simulink model "SGBMDisparityExample_original"  (R2021a)
settings: Solver=FixedStepDiscrete  StartTime=0.0  StopTime=simT  FixedStep=1  RelTol=1e-3
PreLoadFcn:
  | DL128 = Simulink.Variant('disparityLevels==128');
  | 
  | DLnot128 = Simulink.Variant('disparityLevels ~= 128');
  | 
  | disparityLevels = 64;
  | 
  | imgRowSize = 480;
  | 
  | imgColSize = 640;
  | 
  | P2 = 200; % Smoothness Penalty Large
  | P1 = 15;  % Smoothness Penalty Small
  | 
  | disparityFactor = 16;
  | 
  | uniquenessRatio = 5;
  | 
  | p = imgColSize - 1;
  | q = imgRowSize * imgColSize -1;
  | r = imgColSize - disparityLevels -1;
  | s = (imgRowSize*(imgColSize-disparityLevels))-1;
  | 
  | simT = 800*525
  | 
  | dtGain = 4;
InitFcn:
  | DL128 = Simulink.Variant('disparityLevels==128');
  | 
  | DLnot128 = Simulink.Variant('disparityLevels ~= 128');
  | 
  | img = imread(get_param('SGBMDisparityExample/leftImage','FileName'));
  | 
  | [imgRowSize, imgColSize] = size(img);
  | 
  | P2 = 200; % Smoothness Penalty Large
  | P1 = 15;  % Smoothness Penalty Small
  | 
  | disparityFactor = 16;
  | 
  | uniquenessRatio = str2num(get_param('SGBMDisparityExample/SGBMHDLAlgorithm','UT'));
  | 
  | disparityLevels = str2num(get_param('SGBMDisparityExample/SGBMHDLAlgorithm','DL'));
  | 
  | p = imgColSize - 1;
  | q = imgRowSize * imgColSize -1;
  | r = imgColSize - disparityLevels -1;
  | s = (imgRowSize*(imgColSize-disparityLevels))-1;
  | 
  | if imgRowSize == 720 && imgColSize == 1280
  | simT = 1650*750;
  | elseif imgRowSize == 540 && imgColSize == 960
  | simT = 1050*600;
  | elseif imgRowSize == 480 && imgColSize == 640
  | simT = 800*525;
  | end
  | 
  | if imgRowSize == 720 && imgColSize == 1280
  | dtGain = 2;
  | elseif imgRowSize == 540 && imgColSize == 960
  | dtGain = 2.6;
  | elseif imgRowSize == 480 && imgColSize == 640
  | dtGain = 4;
  | end
libraries: simulink x331, hdlsllib x105, visionhdlutilities x10, visionhdlio x4, visionsources x3
(part 5 of 6)

== system SGBMDisparityExample_original/SGBMHDLAlgorithm/MatchingCost/CensusTransform1/validLogic/pixelBusGenerator ==
  validIn : Inport
  Horizontal : hdlsllib/Sources/HDL Counter  CountType=Count limited  CountInit=0  CountStep=1  CountMax=hEnd  CountFromType=Initial value  CountFrom=0  CountResetPort=off  CountLoadPort=off  CountEnbPort=on  CountDirPort=off  CountHitOutputPort=off  CountDataType=Unsigned  CountWordLen=ceil(log2(hEnd))  CountFracLen=0  CountSampTime=1
  Logical Operator{3..6} (4 alike) : Logic  AllPortsSameDT=off  OutDataTypeStr=boolean
  Pixel Control Bus Creator : visionhdlutilities/Pixel Control Bus Creator
      settings: SourceProductBaseCode=VT
  Vertical : hdlsllib/Sources/HDL Counter  CountType=Count limited  CountInit=0  CountStep=1  CountMax=vEnd  CountFromType=Initial value  CountFrom=0  CountResetPort=off  CountLoadPort=off  CountEnbPort=on  CountDirPort=off  CountHitOutputPort=off  CountDataType=Unsigned  CountWordLen=ceil(log2(vEnd))  CountFracLen=0  CountSampTime=1
  hEnd : simulink/Logic and Bit Operations/Compare To Constant  relop===  const=hEnd  OutDataTypeStr=boolean
  hStart : simulink/Logic and Bit Operations/Compare To Constant  relop===  const=0  OutDataTypeStr=boolean
  vEnd : simulink/Logic and Bit Operations/Compare To Constant  relop===  const=vEnd  OutDataTypeStr=boolean
  vStart : simulink/Logic and Bit Operations/Compare To Constant  relop===  const=0  OutDataTypeStr=boolean
  busOut : Outport  VectorParamsAs1DForOutWhenUnconnected=off
  wires:
  validIn/1 -> Pixel Control Bus Creator/5, Vertical/1, Logical Operator4/1, Logical Operator5/1, Logical Operator6/1, Logical Operator3/1, Horizontal/1
  Horizontal/1 -> hEnd/1, hStart/1
  hEnd/1 -> Logical Operator4/2
  Vertical/1 -> vStart/1, vEnd/1
  vStart/1 -> Logical Operator5/2
  vEnd/1 -> Logical Operator6/2
  Logical Operator5/1 -> Pixel Control Bus Creator/3
  Logical Operator3/1 -> Pixel Control Bus Creator/1
  Logical Operator4/1 -> Pixel Control Bus Creator/2
  hStart/1 -> Logical Operator3/2
  Logical Operator6/1 -> Pixel Control Bus Creator/4
  Pixel Control Bus Creator/1 -> busOut/1

== system SGBMDisparityExample_original/SGBMHDLAlgorithm/MatchingCost/CensusTransform1/zeroPadding/FIFO ==
  dataIn : Inport
  Push : Inport  Port=2
  Pop : Inport  Port=3
  Reset : Inport  Port=4
  EmpltyFlag : RelationalOperator  Operator===  OutDataTypeStr=boolean  RndMeth=Nearest
  HDL Counter : hdlsllib/Sources/HDL Counter  CountType=Count limited  CountInit=0  CountStep=1  CountMax=((imgRowSize+6)*(imgColSize+8))-(imgRowSize*imgColSize)  CountFromType=Initial value  CountFrom=0  CountResetPort=on  CountLoadPort=off  CountEnbPort=on  CountDirPort=off  CountHitOutputPort=off  CountDataType=Unsigned  CountWordLen=ceil(log2(((imgRowSize+6)*(imgColSize+8))-(imgRowSize*imgColSize)))  CountFracLen=0  CountSampTime=1
  HDL Counter1 : hdlsllib/Sources/HDL Counter  CountType=Count limited  CountInit=0  CountStep=1  CountMax=((imgRowSize+6)*(imgColSize+8))-(imgRowSize*imgColSize)  CountFromType=Initial value  CountFrom=0  CountResetPort=on  CountLoadPort=off  CountEnbPort=on  CountDirPort=off  CountHitOutputPort=off  CountDataType=Unsigned  CountWordLen=ceil(log2(((imgRowSize+6)*(imgColSize+8))-(imgRowSize*imgColSize)))  CountFracLen=0  CountSampTime=1
  Simple Dual Port RAM : hdlsllib/HDL RAMs/Simple Dual Port RAM  ram_size=ceil(log2(((imgRowSize+6)*(imgColSize+8))-(imgRowSize*imgColSize)))
      settings: SourceProductBaseCode=SL
  dataOut : Outport  VectorParamsAs1DForOutWhenUnconnected=off
  empty : Outport  Port=2  VectorParamsAs1DForOutWhenUnconnected=off
  wires:
  HDL Counter1/1 -> EmpltyFlag/2, Simple Dual Port RAM/4
  Pop/1 -> HDL Counter1/2
  HDL Counter/1 -> EmpltyFlag/1, Simple Dual Port RAM/2
  Push/1 -> HDL Counter/2, Simple Dual Port RAM/3
  dataIn/1 -> Simple Dual Port RAM/1
  Simple Dual Port RAM/1 -> dataOut/1
  EmpltyFlag/1 -> empty/1
  Reset/1 -> HDL Counter1/1, HDL Counter/1

== system SGBMDisparityExample_original/SGBMHDLAlgorithm/MatchingCost/CensusTransform1/zeroPadding/popSubsystem ==
  enable : Inport
  reset : Inport  Port=2
  Enable : EnablePort
  CC : simulink/Logic and Bit Operations/Compare To Constant  relop===  const=imgColSize+7  OutDataTypeStr=boolean
  CC1 : simulink/Logic and Bit Operations/Compare To Constant  relop=>=  const=3  OutDataTypeStr=boolean
  CC2 : simulink/Logic and Bit Operations/Compare To Constant  relop=>=  const=4  OutDataTypeStr=boolean
  CC3 : simulink/Logic and Bit Operations/Compare To Constant  relop=<  const=imgColSize+4  OutDataTypeStr=boolean
  CC4 : simulink/Logic and Bit Operations/Compare To Constant  relop=<  const=imgRowSize + 3  OutDataTypeStr=boolean
  CC6 : simulink/Logic and Bit Operations/Compare To Constant  relop===  const=imgRowSize + 5  OutDataTypeStr=boolean
  CC8 : simulink/Logic and Bit Operations/Compare To Constant  relop=>=  const=imgRowSize+2  OutDataTypeStr=boolean
  HDLC1 : hdlsllib/Sources/HDL Counter  CountType=Count limited  CountInit=0  CountStep=1  CountMax=imgColSize+7  CountFromType=Initial value  CountFrom=0  CountResetPort=on  CountLoadPort=off  CountEnbPort=on  CountDirPort=off  CountHitOutputPort=off  CountDataType=Unsigned  CountWordLen=ceil(log2(imgColSize+7))  CountFracLen=0  CountSampTime=1
  HDLC2 : hdlsllib/Sources/HDL Counter  CountType=Count limited  CountInit=0  CountStep=1  CountMax=imgRowSize+6  CountFromType=Initial value  CountFrom=0  CountResetPort=on  CountLoadPort=off  CountEnbPort=on  CountDirPort=off  CountHitOutputPort=off  CountDataType=Unsigned  CountWordLen=ceil(log2(imgRowSize+6))  CountFracLen=0  CountSampTime=1
  LO2 : Logic  Inputs=4  AllPortsSameDT=off  OutDataTypeStr=boolean
  LO4 : Logic  AllPortsSameDT=off  OutDataTypeStr=boolean
  done : Outport  InitialOutput=0  VectorParamsAs1DForOutWhenUnconnected=off
  pop : Outport  Port=2  InitialOutput=0  VectorParamsAs1DForOutWhenUnconnected=off
  lastRowOut : Outport  Port=3  InitialOutput=0  VectorParamsAs1DForOutWhenUnconnected=off
  wires:
  HDLC2/1 -> CC1/1, CC6/1, CC8/1, CC4/1
  CC4/1 -> LO2/2
  HDLC1/1 -> CC3/1, CC2/1, CC/1
  CC/1 -> HDLC2/2, LO4/1
  CC2/1 -> LO2/3
  CC3/1 -> LO2/4
  CC1/1 -> LO2/1
  CC6/1 -> LO4/2
  LO2/1 -> pop/1
  CC8/1 -> lastRowOut/1
  enable/1 -> HDLC1/2
  LO4/1 -> done/1
  reset/1 -> HDLC2/1, HDLC1/1

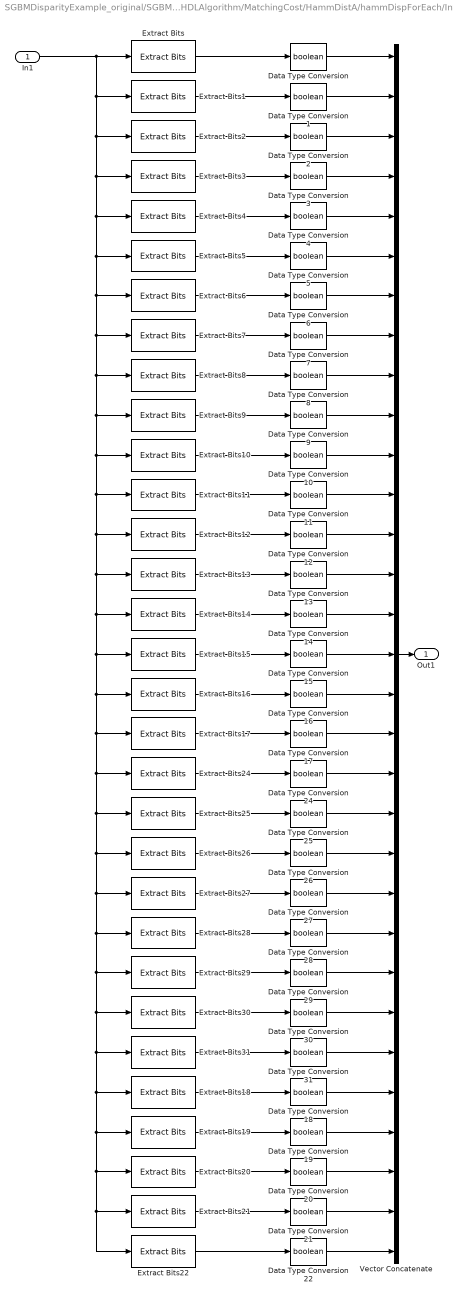
== system SGBMDisparityExample_original/SGBMHDLAlgorithm/MatchingCost/HammDistA/hammDispForEach/Int2Bin1 ==
  In1 : Inport
  Data Type Conversion{,1..22,24..31} (31 alike) : DataTypeConversion  OutDataTypeStr=boolean
  Extract Bits : simulink/Logic and Bit Operations/Extract Bits  bitsToExtract=Range of bits  numBits=8  bitIdxRange=[30]  outScalingMode=Treat bit field as an integer
  Extract Bits1 : simulink/Logic and Bit Operations/Extract Bits  bitsToExtract=Range of bits  numBits=8  bitIdxRange=[29]  outScalingMode=Treat bit field as an integer
  Extract Bits10 : simulink/Logic and Bit Operations/Extract Bits  bitsToExtract=Range of bits  numBits=8  bitIdxRange=[20]  outScalingMode=Preserve fixed-point scaling
  Extract Bits11 : simulink/Logic and Bit Operations/Extract Bits  bitsToExtract=Range of bits  numBits=8  bitIdxRange=[19]  outScalingMode=Preserve fixed-point scaling
  Extract Bits12 : simulink/Logic and Bit Operations/Extract Bits  bitsToExtract=Range of bits  numBits=8  bitIdxRange=[18]  outScalingMode=Preserve fixed-point scaling
  Extract Bits13 : simulink/Logic and Bit Operations/Extract Bits  bitsToExtract=Range of bits  numBits=8  bitIdxRange=[17]  outScalingMode=Preserve fixed-point scaling
  Extract Bits14 : simulink/Logic and Bit Operations/Extract Bits  bitsToExtract=Range of bits  numBits=8  bitIdxRange=[16]  outScalingMode=Preserve fixed-point scaling
  Extract Bits15 : simulink/Logic and Bit Operations/Extract Bits  bitsToExtract=Range of bits  numBits=8  bitIdxRange=[15]  outScalingMode=Preserve fixed-point scaling
  Extract Bits16 : simulink/Logic and Bit Operations/Extract Bits  bitsToExtract=Range of bits  numBits=8  bitIdxRange=[14]  outScalingMode=Preserve fixed-point scaling
  Extract Bits17 : simulink/Logic and Bit Operations/Extract Bits  bitsToExtract=Range of bits  numBits=8  bitIdxRange=[13]  outScalingMode=Preserve fixed-point scaling
  Extract Bits18 : simulink/Logic and Bit Operations/Extract Bits  bitsToExtract=Range of bits  numBits=8  bitIdxRange=[4]  outScalingMode=Preserve fixed-point scaling
  Extract Bits19 : simulink/Logic and Bit Operations/Extract Bits  bitsToExtract=Range of bits  numBits=8  bitIdxRange=[3]  outScalingMode=Preserve fixed-point scaling
  Extract Bits2 : simulink/Logic and Bit Operations/Extract Bits  bitsToExtract=Range of bits  numBits=8  bitIdxRange=[28]  outScalingMode=Treat bit field as an integer
  Extract Bits20 : simulink/Logic and Bit Operations/Extract Bits  bitsToExtract=Range of bits  numBits=8  bitIdxRange=[2]  outScalingMode=Preserve fixed-point scaling
  Extract Bits21 : simulink/Logic and Bit Operations/Extract Bits  bitsToExtract=Range of bits  numBits=8  bitIdxRange=[1]  outScalingMode=Preserve fixed-point scaling
  Extract Bits22 : simulink/Logic and Bit Operations/Extract Bits  bitsToExtract=Range of bits  numBits=8  bitIdxRange=[0]  outScalingMode=Preserve fixed-point scaling
  Extract Bits24 : simulink/Logic and Bit Operations/Extract Bits  bitsToExtract=Range of bits  numBits=8  bitIdxRange=[12]  outScalingMode=Preserve fixed-point scaling
  Extract Bits25 : simulink/Logic and Bit Operations/Extract Bits  bitsToExtract=Range of bits  numBits=8  bitIdxRange=[11]  outScalingMode=Preserve fixed-point scaling
  Extract Bits26 : simulink/Logic and Bit Operations/Extract Bits  bitsToExtract=Range of bits  numBits=8  bitIdxRange=[10]  outScalingMode=Preserve fixed-point scaling
  Extract Bits27 : simulink/Logic and Bit Operations/Extract Bits  bitsToExtract=Range of bits  numBits=8  bitIdxRange=[9]  outScalingMode=Preserve fixed-point scaling
  Extract Bits28 : simulink/Logic and Bit Operations/Extract Bits  bitsToExtract=Range of bits  numBits=8  bitIdxRange=[8]  outScalingMode=Preserve fixed-point scaling
  Extract Bits29 : simulink/Logic and Bit Operations/Extract Bits  bitsToExtract=Range of bits  numBits=8  bitIdxRange=[7]  outScalingMode=Preserve fixed-point scaling
  Extract Bits3 : simulink/Logic and Bit Operations/Extract Bits  bitsToExtract=Range of bits  numBits=8  bitIdxRange=[27]  outScalingMode=Treat bit field as an integer
  Extract Bits30 : simulink/Logic and Bit Operations/Extract Bits  bitsToExtract=Range of bits  numBits=8  bitIdxRange=[6]  outScalingMode=Preserve fixed-point scaling
  Extract Bits31 : simulink/Logic and Bit Operations/Extract Bits  bitsToExtract=Range of bits  numBits=8  bitIdxRange=[5]  outScalingMode=Preserve fixed-point scaling
  Extract Bits4 : simulink/Logic and Bit Operations/Extract Bits  bitsToExtract=Range of bits  numBits=8  bitIdxRange=[26]  outScalingMode=Treat bit field as an integer
  Extract Bits5 : simulink/Logic and Bit Operations/Extract Bits  bitsToExtract=Range of bits  numBits=8  bitIdxRange=[25]  outScalingMode=Treat bit field as an integer
  Extract Bits6 : simulink/Logic and Bit Operations/Extract Bits  bitsToExtract=Range of bits  numBits=8  bitIdxRange=[24]  outScalingMode=Treat bit field as an integer
  Extract Bits7 : simulink/Logic and Bit Operations/Extract Bits  bitsToExtract=Range of bits  numBits=8  bitIdxRange=[23]  outScalingMode=Treat bit field as an integer
  Extract Bits8 : simulink/Logic and Bit Operations/Extract Bits  bitsToExtract=Range of bits  numBits=8  bitIdxRange=[22]  outScalingMode=Preserve fixed-point scaling
  Extract Bits9 : simulink/Logic and Bit Operations/Extract Bits  bitsToExtract=Range of bits  numBits=8  bitIdxRange=[21]  outScalingMode=Preserve fixed-point scaling
  Vector Concatenate : Concatenate  NumInputs=31
  Out1 : Outport  VectorParamsAs1DForOutWhenUnconnected=off
  wires:
  Extract Bits6/1 -> Data Type Conversion6/1
  Extract Bits8/1 -> Data Type Conversion8/1
  Extract Bits1/1 -> Data Type Conversion1/1
  Extract Bits2/1 -> Data Type Conversion2/1
  Extract Bits9/1 -> Data Type Conversion9/1
  Extract Bits10/1 -> Data Type Conversion10/1
  Extract Bits3/1 -> Data Type Conversion3/1
  Extract Bits4/1 -> Data Type Conversion4/1
  Extract Bits11/1 -> Data Type Conversion11/1
  Extract Bits12/1 -> Data Type Conversion12/1
  Extract Bits13/1 -> Data Type Conversion13/1
  Extract Bits/1 -> Data Type Conversion/1
  Extract Bits7/1 -> Data Type Conversion7/1
  Extract Bits5/1 -> Data Type Conversion5/1
  Extract Bits31/1 -> Data Type Conversion31/1
  Extract Bits26/1 -> Data Type Conversion26/1
  Extract Bits18/1 -> Data Type Conversion18/1
  Extract Bits14/1 -> Data Type Conversion14/1
  Extract Bits21/1 -> Data Type Conversion21/1
  Extract Bits16/1 -> Data Type Conversion16/1
  Extract Bits25/1 -> Data Type Conversion25/1
  Extract Bits27/1 -> Data Type Conversion27/1
  Extract Bits30/1 -> Data Type Conversion30/1
  Extract Bits20/1 -> Data Type Conversion20/1
  Extract Bits28/1 -> Data Type Conversion28/1
  Extract Bits22/1 -> Data Type Conversion22/1
  Extract Bits24/1 -> Data Type Conversion24/1
  Extract Bits19/1 -> Data Type Conversion19/1
  Extract Bits15/1 -> Data Type Conversion15/1
  Extract Bits17/1 -> Data Type Conversion17/1
  Extract Bits29/1 -> Data Type Conversion29/1
  Vector Concatenate/1 -> Out1/1
  In1/1 -> Extract Bits/1, Extract Bits1/1, Extract Bits2/1, Extract Bits3/1, Extract Bits4/1, Extract Bits5/1, Extract Bits6/1, Extract Bits7/1, Extract Bits8/1, Extract Bits9/1, Extract Bits10/1, Extract Bits11/1, Extract Bits12/1, Extract Bits13/1, Extract Bits14/1, Extract Bits15/1, Extract Bits16/1, Extract Bits17/1, Extract Bits24/1, Extract Bits25/1, Extract Bits26/1, Extract Bits27/1, Extract Bits28/1, Extract Bits29/1, Extract Bits30/1, Extract Bits31/1, Extract Bits18/1, Extract Bits19/1, Extract Bits20/1, Extract Bits21/1, Extract Bits22/1
  Data Type Conversion/1 -> Vector Concatenate/1
  Data Type Conversion1/1 -> Vector Concatenate/2
  Data Type Conversion2/1 -> Vector Concatenate/3
  Data Type Conversion3/1 -> Vector Concatenate/4
  Data Type Conversion4/1 -> Vector Concatenate/5
  Data Type Conversion7/1 -> Vector Concatenate/8
  Data Type Conversion6/1 -> Vector Concatenate/7
  Data Type Conversion5/1 -> Vector Concatenate/6
  Data Type Conversion8/1 -> Vector Concatenate/9
  Data Type Conversion10/1 -> Vector Concatenate/11
  Data Type Conversion9/1 -> Vector Concatenate/10
  Data Type Conversion11/1 -> Vector Concatenate/12
  Data Type Conversion14/1 -> Vector Concatenate/15
  Data Type Conversion12/1 -> Vector Concatenate/13
  Data Type Conversion13/1 -> Vector Concatenate/14
  Data Type Conversion15/1 -> Vector Concatenate/16
  Data Type Conversion20/1 -> Vector Concatenate/29
  Data Type Conversion21/1 -> Vector Concatenate/30
  Data Type Conversion24/1 -> Vector Concatenate/19
  Data Type Conversion22/1 -> Vector Concatenate/31
  Data Type Conversion27/1 -> Vector Concatenate/22
  Data Type Conversion26/1 -> Vector Concatenate/21
  Data Type Conversion25/1 -> Vector Concatenate/20
  Data Type Conversion29/1 -> Vector Concatenate/24
  Data Type Conversion28/1 -> Vector Concatenate/23
  Data Type Conversion30/1 -> Vector Concatenate/25
  Data Type Conversion31/1 -> Vector Concatenate/26
  Data Type Conversion16/1 -> Vector Concatenate/17
  Data Type Conversion17/1 -> Vector Concatenate/18
  Data Type Conversion19/1 -> Vector Concatenate/28
  Data Type Conversion18/1 -> Vector Concatenate/27

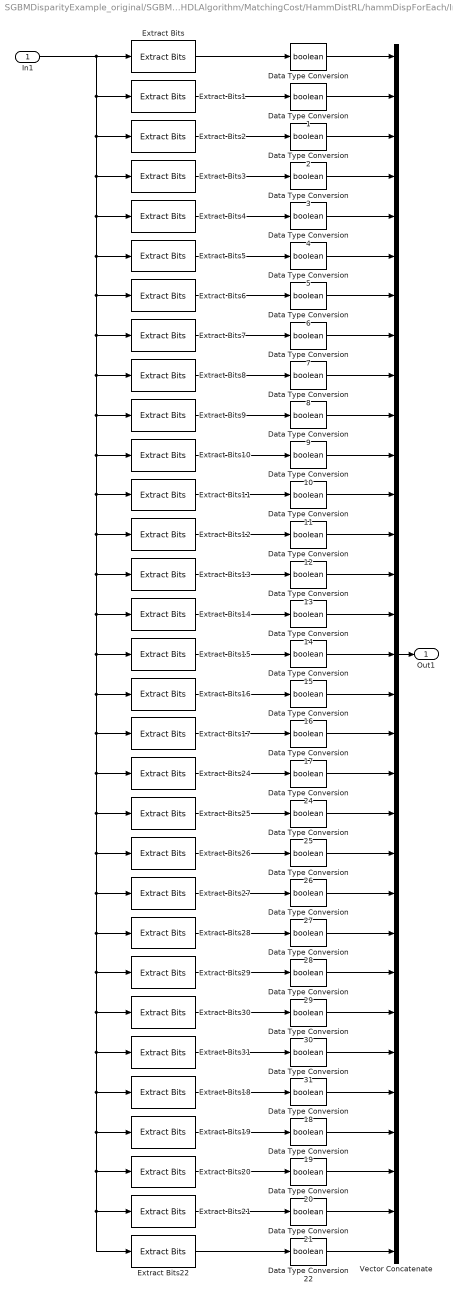
== system SGBMDisparityExample_original/SGBMHDLAlgorithm/MatchingCost/HammDistRL/hammDispForEach/Int2Bin1 ==
  In1 : Inport
  Data Type Conversion{,1..22,24..31} (31 alike) : DataTypeConversion  OutDataTypeStr=boolean
  Extract Bits : simulink/Logic and Bit Operations/Extract Bits  bitsToExtract=Range of bits  numBits=8  bitIdxRange=[30]  outScalingMode=Treat bit field as an integer
  Extract Bits1 : simulink/Logic and Bit Operations/Extract Bits  bitsToExtract=Range of bits  numBits=8  bitIdxRange=[29]  outScalingMode=Treat bit field as an integer
  Extract Bits10 : simulink/Logic and Bit Operations/Extract Bits  bitsToExtract=Range of bits  numBits=8  bitIdxRange=[20]  outScalingMode=Preserve fixed-point scaling
  Extract Bits11 : simulink/Logic and Bit Operations/Extract Bits  bitsToExtract=Range of bits  numBits=8  bitIdxRange=[19]  outScalingMode=Preserve fixed-point scaling
  Extract Bits12 : simulink/Logic and Bit Operations/Extract Bits  bitsToExtract=Range of bits  numBits=8  bitIdxRange=[18]  outScalingMode=Preserve fixed-point scaling
  Extract Bits13 : simulink/Logic and Bit Operations/Extract Bits  bitsToExtract=Range of bits  numBits=8  bitIdxRange=[17]  outScalingMode=Preserve fixed-point scaling
  Extract Bits14 : simulink/Logic and Bit Operations/Extract Bits  bitsToExtract=Range of bits  numBits=8  bitIdxRange=[16]  outScalingMode=Preserve fixed-point scaling
  Extract Bits15 : simulink/Logic and Bit Operations/Extract Bits  bitsToExtract=Range of bits  numBits=8  bitIdxRange=[15]  outScalingMode=Preserve fixed-point scaling
  Extract Bits16 : simulink/Logic and Bit Operations/Extract Bits  bitsToExtract=Range of bits  numBits=8  bitIdxRange=[14]  outScalingMode=Preserve fixed-point scaling
  Extract Bits17 : simulink/Logic and Bit Operations/Extract Bits  bitsToExtract=Range of bits  numBits=8  bitIdxRange=[13]  outScalingMode=Preserve fixed-point scaling
  Extract Bits18 : simulink/Logic and Bit Operations/Extract Bits  bitsToExtract=Range of bits  numBits=8  bitIdxRange=[4]  outScalingMode=Preserve fixed-point scaling
  Extract Bits19 : simulink/Logic and Bit Operations/Extract Bits  bitsToExtract=Range of bits  numBits=8  bitIdxRange=[3]  outScalingMode=Preserve fixed-point scaling
  Extract Bits2 : simulink/Logic and Bit Operations/Extract Bits  bitsToExtract=Range of bits  numBits=8  bitIdxRange=[28]  outScalingMode=Treat bit field as an integer
  Extract Bits20 : simulink/Logic and Bit Operations/Extract Bits  bitsToExtract=Range of bits  numBits=8  bitIdxRange=[2]  outScalingMode=Preserve fixed-point scaling
  Extract Bits21 : simulink/Logic and Bit Operations/Extract Bits  bitsToExtract=Range of bits  numBits=8  bitIdxRange=[1]  outScalingMode=Preserve fixed-point scaling
  Extract Bits22 : simulink/Logic and Bit Operations/Extract Bits  bitsToExtract=Range of bits  numBits=8  bitIdxRange=[0]  outScalingMode=Preserve fixed-point scaling
  Extract Bits24 : simulink/Logic and Bit Operations/Extract Bits  bitsToExtract=Range of bits  numBits=8  bitIdxRange=[12]  outScalingMode=Preserve fixed-point scaling
  Extract Bits25 : simulink/Logic and Bit Operations/Extract Bits  bitsToExtract=Range of bits  numBits=8  bitIdxRange=[11]  outScalingMode=Preserve fixed-point scaling
  Extract Bits26 : simulink/Logic and Bit Operations/Extract Bits  bitsToExtract=Range of bits  numBits=8  bitIdxRange=[10]  outScalingMode=Preserve fixed-point scaling
  Extract Bits27 : simulink/Logic and Bit Operations/Extract Bits  bitsToExtract=Range of bits  numBits=8  bitIdxRange=[9]  outScalingMode=Preserve fixed-point scaling
  Extract Bits28 : simulink/Logic and Bit Operations/Extract Bits  bitsToExtract=Range of bits  numBits=8  bitIdxRange=[8]  outScalingMode=Preserve fixed-point scaling
  Extract Bits29 : simulink/Logic and Bit Operations/Extract Bits  bitsToExtract=Range of bits  numBits=8  bitIdxRange=[7]  outScalingMode=Preserve fixed-point scaling
  Extract Bits3 : simulink/Logic and Bit Operations/Extract Bits  bitsToExtract=Range of bits  numBits=8  bitIdxRange=[27]  outScalingMode=Treat bit field as an integer
  Extract Bits30 : simulink/Logic and Bit Operations/Extract Bits  bitsToExtract=Range of bits  numBits=8  bitIdxRange=[6]  outScalingMode=Preserve fixed-point scaling
  Extract Bits31 : simulink/Logic and Bit Operations/Extract Bits  bitsToExtract=Range of bits  numBits=8  bitIdxRange=[5]  outScalingMode=Preserve fixed-point scaling
  Extract Bits4 : simulink/Logic and Bit Operations/Extract Bits  bitsToExtract=Range of bits  numBits=8  bitIdxRange=[26]  outScalingMode=Treat bit field as an integer
  Extract Bits5 : simulink/Logic and Bit Operations/Extract Bits  bitsToExtract=Range of bits  numBits=8  bitIdxRange=[25]  outScalingMode=Treat bit field as an integer
  Extract Bits6 : simulink/Logic and Bit Operations/Extract Bits  bitsToExtract=Range of bits  numBits=8  bitIdxRange=[24]  outScalingMode=Treat bit field as an integer
  Extract Bits7 : simulink/Logic and Bit Operations/Extract Bits  bitsToExtract=Range of bits  numBits=8  bitIdxRange=[23]  outScalingMode=Treat bit field as an integer
  Extract Bits8 : simulink/Logic and Bit Operations/Extract Bits  bitsToExtract=Range of bits  numBits=8  bitIdxRange=[22]  outScalingMode=Preserve fixed-point scaling
  Extract Bits9 : simulink/Logic and Bit Operations/Extract Bits  bitsToExtract=Range of bits  numBits=8  bitIdxRange=[21]  outScalingMode=Preserve fixed-point scaling
  Vector Concatenate : Concatenate  NumInputs=31
  Out1 : Outport  VectorParamsAs1DForOutWhenUnconnected=off
  wires:
  Extract Bits6/1 -> Data Type Conversion6/1
  Extract Bits8/1 -> Data Type Conversion8/1
  Extract Bits1/1 -> Data Type Conversion1/1
  Extract Bits2/1 -> Data Type Conversion2/1
  Extract Bits9/1 -> Data Type Conversion9/1
  Extract Bits10/1 -> Data Type Conversion10/1
  Extract Bits3/1 -> Data Type Conversion3/1
  Extract Bits4/1 -> Data Type Conversion4/1
  Extract Bits11/1 -> Data Type Conversion11/1
  Extract Bits12/1 -> Data Type Conversion12/1
  Extract Bits13/1 -> Data Type Conversion13/1
  Extract Bits/1 -> Data Type Conversion/1
  Extract Bits7/1 -> Data Type Conversion7/1
  Extract Bits5/1 -> Data Type Conversion5/1
  Extract Bits31/1 -> Data Type Conversion31/1
  Extract Bits26/1 -> Data Type Conversion26/1
  Extract Bits18/1 -> Data Type Conversion18/1
  Extract Bits14/1 -> Data Type Conversion14/1
  Extract Bits21/1 -> Data Type Conversion21/1
  Extract Bits16/1 -> Data Type Conversion16/1
  Extract Bits25/1 -> Data Type Conversion25/1
  Extract Bits27/1 -> Data Type Conversion27/1
  Extract Bits30/1 -> Data Type Conversion30/1
  Extract Bits20/1 -> Data Type Conversion20/1
  Extract Bits28/1 -> Data Type Conversion28/1
  Extract Bits22/1 -> Data Type Conversion22/1
  Extract Bits24/1 -> Data Type Conversion24/1
  Extract Bits19/1 -> Data Type Conversion19/1
  Extract Bits15/1 -> Data Type Conversion15/1
  Extract Bits17/1 -> Data Type Conversion17/1
  Extract Bits29/1 -> Data Type Conversion29/1
  Vector Concatenate/1 -> Out1/1
  In1/1 -> Extract Bits/1, Extract Bits1/1, Extract Bits2/1, Extract Bits3/1, Extract Bits4/1, Extract Bits5/1, Extract Bits6/1, Extract Bits7/1, Extract Bits8/1, Extract Bits9/1, Extract Bits10/1, Extract Bits11/1, Extract Bits12/1, Extract Bits13/1, Extract Bits14/1, Extract Bits15/1, Extract Bits16/1, Extract Bits17/1, Extract Bits24/1, Extract Bits25/1, Extract Bits26/1, Extract Bits27/1, Extract Bits28/1, Extract Bits29/1, Extract Bits30/1, Extract Bits31/1, Extract Bits18/1, Extract Bits19/1, Extract Bits20/1, Extract Bits21/1, Extract Bits22/1
  Data Type Conversion/1 -> Vector Concatenate/1
  Data Type Conversion1/1 -> Vector Concatenate/2
  Data Type Conversion2/1 -> Vector Concatenate/3
  Data Type Conversion3/1 -> Vector Concatenate/4
  Data Type Conversion4/1 -> Vector Concatenate/5
  Data Type Conversion7/1 -> Vector Concatenate/8
  Data Type Conversion6/1 -> Vector Concatenate/7
  Data Type Conversion5/1 -> Vector Concatenate/6
  Data Type Conversion8/1 -> Vector Concatenate/9
  Data Type Conversion10/1 -> Vector Concatenate/11
  Data Type Conversion9/1 -> Vector Concatenate/10
  Data Type Conversion11/1 -> Vector Concatenate/12
  Data Type Conversion14/1 -> Vector Concatenate/15
  Data Type Conversion12/1 -> Vector Concatenate/13
  Data Type Conversion13/1 -> Vector Concatenate/14
  Data Type Conversion15/1 -> Vector Concatenate/16
  Data Type Conversion20/1 -> Vector Concatenate/29
  Data Type Conversion21/1 -> Vector Concatenate/30
  Data Type Conversion24/1 -> Vector Concatenate/19
  Data Type Conversion22/1 -> Vector Concatenate/31
  Data Type Conversion27/1 -> Vector Concatenate/22
  Data Type Conversion26/1 -> Vector Concatenate/21
  Data Type Conversion25/1 -> Vector Concatenate/20
  Data Type Conversion29/1 -> Vector Concatenate/24
  Data Type Conversion28/1 -> Vector Concatenate/23
  Data Type Conversion30/1 -> Vector Concatenate/25
  Data Type Conversion31/1 -> Vector Concatenate/26
  Data Type Conversion16/1 -> Vector Concatenate/17
  Data Type Conversion17/1 -> Vector Concatenate/18
  Data Type Conversion19/1 -> Vector Concatenate/28
  Data Type Conversion18/1 -> Vector Concatenate/27

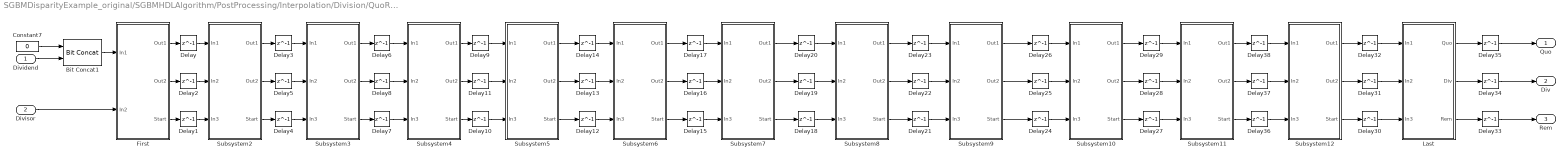
== system SGBMDisparityExample_original/SGBMHDLAlgorithm/PostProcessing/Interpolation/Division/QuoRem ==
  Dividend : Inport
  Divisor : Inport  Port=2
  Bit Concat1 : hdlsllib/Logic and Bit Operations/Bit Concat  numInputs=2
  Constant7 : Constant  Value=0  OutDataTypeStr=fixdt(0,13,0)  SampleTime=-1
  Delay{,1..38} (39 alike) : Delay  DelayLength=1
  First : Subsystem
  Last : Subsystem
  Subsystem10 : Subsystem
  Subsystem11 : Subsystem
  Subsystem12 : Subsystem
  Subsystem2 : Subsystem
  Subsystem3 : Subsystem
  Subsystem4 : Subsystem
  Subsystem5 : Subsystem
  Subsystem6 : Subsystem
  Subsystem7 : Subsystem
  Subsystem8 : Subsystem
  Subsystem9 : Subsystem
  Quo : Outport  VectorParamsAs1DForOutWhenUnconnected=off
  Div : Outport  Port=2  VectorParamsAs1DForOutWhenUnconnected=off
  Rem : Outport  Port=3  VectorParamsAs1DForOutWhenUnconnected=off
  wires:
  Constant7/1 -> Bit Concat1/1
  Dividend/1 -> Bit Concat1/2
  Bit Concat1/1 -> First/1(In1)
  Divisor/1 -> First/2(In2)
  Subsystem12/1(Out1) -> Delay32/1
  Subsystem12/2(Out2) -> Delay31/1
  Last/2(Div) -> Delay34/1
  Last/1(Quo) -> Delay35/1
  Last/3(Rem) -> Delay33/1
  First/1(Out1) -> Delay/1
  First/2(Out2) -> Delay2/1
  First/3(Start) -> Delay1/1
  Subsystem2/2(Out2) -> Delay5/1
  Subsystem2/1(Out1) -> Delay3/1
  Subsystem2/3(Start) -> Delay4/1
  Subsystem4/2(Out2) -> Delay11/1
  Subsystem4/3(Start) -> Delay10/1
  Subsystem4/1(Out1) -> Delay9/1
  Subsystem3/2(Out2) -> Delay8/1
  Subsystem3/1(Out1) -> Delay6/1
  Subsystem3/3(Start) -> Delay7/1
  Subsystem6/2(Out2) -> Delay16/1
  Subsystem6/3(Start) -> Delay15/1
  Subsystem6/1(Out1) -> Delay17/1
  Subsystem8/2(Out2) -> Delay22/1
  Subsystem8/1(Out1) -> Delay23/1
  Subsystem7/2(Out2) -> Delay19/1
  Subsystem7/3(Start) -> Delay18/1
  Subsystem5/2(Out2) -> Delay13/1
  Subsystem7/1(Out1) -> Delay20/1
  Subsystem5/1(Out1) -> Delay14/1
  Subsystem5/3(Start) -> Delay12/1
  Subsystem8/3(Start) -> Delay21/1
  Subsystem9/2(Out2) -> Delay25/1
  Subsystem9/3(Start) -> Delay24/1
  Subsystem10/2(Out2) -> Delay28/1
  Subsystem10/1(Out1) -> Delay29/1
  Subsystem10/3(Start) -> Delay27/1
  Subsystem9/1(Out1) -> Delay26/1
  Subsystem12/3(Start) -> Delay30/1
  Delay/1 -> Subsystem2/1(In1)
  Delay1/1 -> Subsystem2/3(In3)
  Delay2/1 -> Subsystem2/2(In2)
  Delay5/1 -> Subsystem3/2(In2)
  Delay4/1 -> Subsystem3/3(In3)
  Delay3/1 -> Subsystem3/1(In1)
  Delay6/1 -> Subsystem4/1(In1)
  Delay8/1 -> Subsystem4/2(In2)
  Delay7/1 -> Subsystem4/3(In3)
  Delay9/1 -> Subsystem5/1(In1)
  Delay10/1 -> Subsystem5/3(In3)
  Delay11/1 -> Subsystem5/2(In2)
  Delay12/1 -> Subsystem6/3(In3)
  Delay13/1 -> Subsystem6/2(In2)
  Delay14/1 -> Subsystem6/1(In1)
  Delay16/1 -> Subsystem7/2(In2)
  Delay15/1 -> Subsystem7/3(In3)
  Delay17/1 -> Subsystem7/1(In1)
  Delay18/1 -> Subsystem8/3(In3)
  Delay20/1 -> Subsystem8/1(In1)
  Delay19/1 -> Subsystem8/2(In2)
  Delay21/1 -> Subsystem9/3(In3)
  Delay22/1 -> Subsystem9/2(In2)
  Delay23/1 -> Subsystem9/1(In1)
  Delay25/1 -> Subsystem10/2(In2)
  Delay24/1 -> Subsystem10/3(In3)
  Delay26/1 -> Subsystem10/1(In1)
  Delay27/1 -> Subsystem11/3(In3)
  Delay28/1 -> Subsystem11/2(In2)
  Delay29/1 -> Subsystem11/1(In1)
  Delay31/1 -> Last/2(In2)
  Delay30/1 -> Last/3(In3)
  Delay32/1 -> Last/1(In1)
  Delay33/1 -> Rem/1
  Delay34/1 -> Div/1
  Delay35/1 -> Quo/1
  Delay36/1 -> Subsystem12/3(In3)
  Delay38/1 -> Subsystem12/1(In1)
  Delay37/1 -> Subsystem12/2(In2)
  Subsystem11/3(Start) -> Delay36/1
  Subsystem11/1(Out1) -> Delay38/1
  Subsystem11/2(Out2) -> Delay37/1

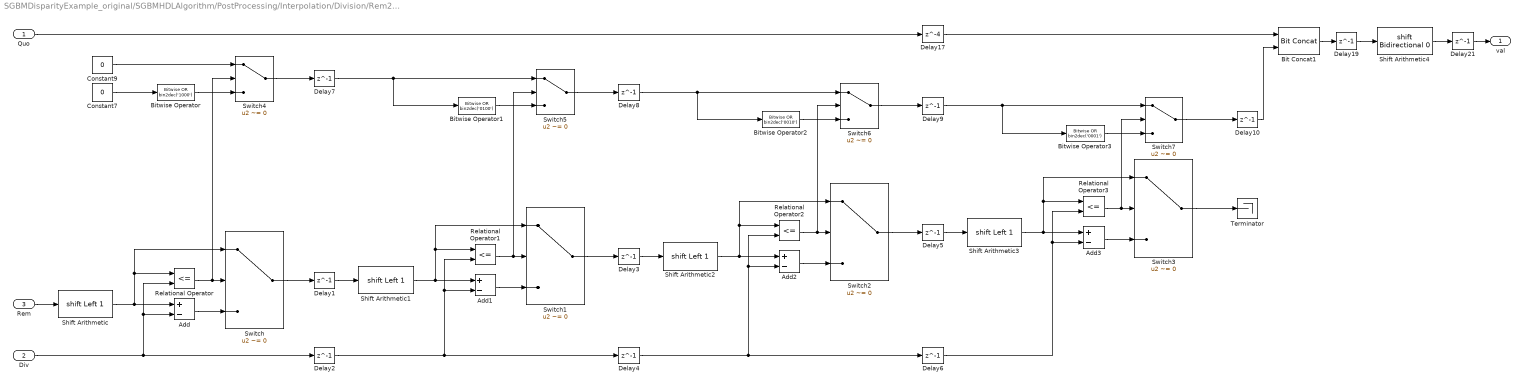
== system SGBMDisparityExample_original/SGBMHDLAlgorithm/PostProcessing/Interpolation/Division/Rem2Bin ==
  Quo : Inport
  Div : Inport  Port=2
  Rem : Inport  Port=3
  Add{,1..3} (4 alike) : Sum  Inputs=+-
  Bit Concat1 : hdlsllib/Logic and Bit Operations/Bit Concat  numInputs=2
  Bitwise Operator : simulink/Logic and Bit Operations/Bitwise Operator  logicop=OR  UseBitMask=on  BitMask=bin2dec('1000')  BitMaskRealWorld=Stored Integer
  Bitwise Operator1 : simulink/Logic and Bit Operations/Bitwise Operator  logicop=OR  UseBitMask=on  BitMask=bin2dec('0100')  BitMaskRealWorld=Stored Integer
  Bitwise Operator2 : simulink/Logic and Bit Operations/Bitwise Operator  logicop=OR  UseBitMask=on  BitMask=bin2dec('0010')  BitMaskRealWorld=Stored Integer
  Bitwise Operator3 : simulink/Logic and Bit Operations/Bitwise Operator  logicop=OR  UseBitMask=on  BitMask=bin2dec('0001')  BitMaskRealWorld=Stored Integer
  Constant7 : Constant  Value=0  OutDataTypeStr=fixdt(0,4,0)  SampleTime=-1
  Constant9 : Constant  Value=0  OutDataTypeStr=fixdt(0,4,0)  SampleTime=-1
  Delay{1..10,19,21} (12 alike) : Delay  DelayLength=1
  Delay17 : Delay  DelayLength=4
  Relational Operator{,1..3} (4 alike) : RelationalOperator  Operator=<=  OutDataTypeStr=boolean  RndMeth=Nearest
  Shift Arithmetic{,1..3} (4 alike) : ArithShift  BitShiftNumber=1  BitShiftDirection=Left
  Shift Arithmetic4 : ArithShift  BinPtShiftNumber=-4
  Switch{,1..7} (8 alike) : Switch  Criteria=u2 ~= 0
  Terminator : Terminator
  val : Outport  VectorParamsAs1DForOutWhenUnconnected=off
  wires:
  Rem/1 -> Shift Arithmetic/1
  Bit Concat1/1 -> Delay19/1
  Quo/1 -> Delay17/1
  Shift Arithmetic4/1 -> Delay21/1
  Delay17/1 -> Bit Concat1/1
  Delay19/1 -> Shift Arithmetic4/1
  Delay21/1 -> val/1
  Shift Arithmetic/1 -> Switch/1, Relational Operator/1, Add/1
  Div/1 -> Delay2/1, Add/2, Relational Operator/2
  Add/1 -> Switch/3
  Relational Operator/1 -> Switch4/2, Switch/2
  Switch/1 -> Delay1/1
  Shift Arithmetic1/1 -> Switch1/1, Relational Operator1/1, Add1/1
  Add1/1 -> Switch1/3
  Delay1/1 -> Shift Arithmetic1/1
  Delay3/1 -> Shift Arithmetic2/1
  Delay2/1 -> Delay4/1, Add1/2, Relational Operator1/2
  Shift Arithmetic2/1 -> Switch2/1, Relational Operator2/1, Add2/1
  Switch1/1 -> Delay3/1
  Add2/1 -> Switch2/3
  Delay4/1 -> Add2/2, Relational Operator2/2, Delay6/1
  Add3/1 -> Switch3/3
  Delay6/1 -> Add3/2, Relational Operator3/2
  Switch3/1 -> Terminator/1
  Switch2/1 -> Delay5/1
  Shift Arithmetic3/1 -> Switch3/1, Relational Operator3/1, Add3/1
  Delay5/1 -> Shift Arithmetic3/1
  Constant7/1 -> Bitwise Operator/1
  Constant9/1 -> Switch4/1
  Bitwise Operator/1 -> Switch4/3
  Bitwise Operator1/1 -> Switch5/3
  Switch4/1 -> Delay7/1
  Relational Operator1/1 -> Switch5/2, Switch1/2
  Delay7/1 -> Bitwise Operator1/1, Switch5/1
  Relational Operator2/1 -> Switch6/2, Switch2/2
  Bitwise Operator2/1 -> Switch6/3
  Delay8/1 -> Bitwise Operator2/1, Switch6/1
  Switch5/1 -> Delay8/1
  Bitwise Operator3/1 -> Switch7/3
  Relational Operator3/1 -> Switch7/2, Switch3/2
  Delay9/1 -> Bitwise Operator3/1, Switch7/1
  Switch6/1 -> Delay9/1
  Switch7/1 -> Delay10/1
  Delay10/1 -> Bit Concat1/2

== system SGBMDisparityExample_original/SGBMHDLAlgorithm/PostProcessing/Interpolation/Minimum_Cost_Index/DL_Vector ==
  note: 1) Add Subsystem or Model blocks as valid variant choices.
      | 2) You cannot connect blocks at this level. At simulation, connectivity is automatically
      | determined, based on the active variant and port name matching.
  In1 : Inport
  DL128 : Subsystem  VariantControl=DL128
  DLnot128 : Subsystem  VariantControl=DLnot128
  Out1 : Outport  VectorParamsAs1DForOutWhenUnconnected=off

== system SGBMDisparityExample_original/SGBMHDLAlgorithm/PostProcessing/Interpolation/Minimum_Cost_Index/For Each Subsystem ==
  In1 : Inport  Partition=on  PartitionDimension=1  PartitionWidth=1  PartitionOffset=0
  In2 : Inport  Port=2  Partition=on  PartitionDimension=1  PartitionWidth=1  PartitionOffset=0
  In3 : Inport  Port=3  Partition=on  PartitionDimension=1  PartitionWidth=1  PartitionOffset=0
  In4 : Inport  Port=4  Partition=on  PartitionDimension=1  PartitionWidth=1  PartitionOffset=0
  In5 : Inport  Port=5  Partition=on  PartitionDimension=1  PartitionWidth=1  PartitionOffset=0
  In6 : Inport  Port=6  Partition=on  PartitionDimension=1  PartitionWidth=1  PartitionOffset=0
  In7 : Inport  Port=7  Partition=on  PartitionDimension=1  PartitionWidth=1  PartitionOffset=0
  In8 : Inport  Port=8  Partition=on  PartitionDimension=1  PartitionWidth=1  PartitionOffset=0
  For Each : ForEach  DisableCoverage=on
  Relational Operator : RelationalOperator  Operator=<=  OutDataTypeStr=boolean  RndMeth=Nearest
  Switch{,1..3} (4 alike) : Switch  Criteria=u2 ~= 0
  Out1 : Outport  ConcatenationDimension=1  VectorParamsAs1DForOutWhenUnconnected=off
  Out2 : Outport  Port=2  ConcatenationDimension=1  VectorParamsAs1DForOutWhenUnconnected=off
  Out3 : Outport  Port=3  ConcatenationDimension=1  VectorParamsAs1DForOutWhenUnconnected=off
  Out4 : Outport  Port=4  ConcatenationDimension=1  VectorParamsAs1DForOutWhenUnconnected=off
  wires:
  In1/1 -> Relational Operator/1, Switch/1
  In2/1 -> Relational Operator/2, Switch/3
  Relational Operator/1 -> Switch3/2, Switch2/2, Switch1/2, Switch/2
  Switch/1 -> Out1/1
  In4/1 -> Switch1/3
  In3/1 -> Switch1/1
  Switch1/1 -> Out2/1
  In6/1 -> Switch2/3
  In5/1 -> Switch2/1
  In8/1 -> Switch3/3
  In7/1 -> Switch3/1
  Switch2/1 -> Out3/1
  Switch3/1 -> Out4/1

== system SGBMDisparityExample_original/SGBMHDLAlgorithm/PostProcessing/Interpolation/Minimum_Cost_Index/For Each Subsystem1 ==
  In1 : Inport  Partition=on  PartitionDimension=1  PartitionWidth=1  PartitionOffset=0
  In2 : Inport  Port=2  Partition=on  PartitionDimension=1  PartitionWidth=1  PartitionOffset=0
  In3 : Inport  Port=3  Partition=on  PartitionDimension=1  PartitionWidth=1  PartitionOffset=0
  In4 : Inport  Port=4  Partition=on  PartitionDimension=1  PartitionWidth=1  PartitionOffset=0
  In5 : Inport  Port=5  Partition=on  PartitionDimension=1  PartitionWidth=1  PartitionOffset=0
  In6 : Inport  Port=6  Partition=on  PartitionDimension=1  PartitionWidth=1  PartitionOffset=0
  In7 : Inport  Port=7  Partition=on  PartitionDimension=1  PartitionWidth=1  PartitionOffset=0
  In8 : Inport  Port=8  Partition=on  PartitionDimension=1  PartitionWidth=1  PartitionOffset=0
  For Each : ForEach  DisableCoverage=on
  Relational Operator : RelationalOperator  Operator=<=  OutDataTypeStr=boolean  RndMeth=Nearest
  Switch{,1..3} (4 alike) : Switch  Criteria=u2 ~= 0
  Out1 : Outport  ConcatenationDimension=1  VectorParamsAs1DForOutWhenUnconnected=off
  Out2 : Outport  Port=2  ConcatenationDimension=1  VectorParamsAs1DForOutWhenUnconnected=off
  Out3 : Outport  Port=3  ConcatenationDimension=1  VectorParamsAs1DForOutWhenUnconnected=off
  Out4 : Outport  Port=4  ConcatenationDimension=1  VectorParamsAs1DForOutWhenUnconnected=off
  wires:
  In1/1 -> Relational Operator/1, Switch/1
  In2/1 -> Relational Operator/2, Switch/3
  Relational Operator/1 -> Switch3/2, Switch2/2, Switch1/2, Switch/2
  Switch/1 -> Out1/1
  In4/1 -> Switch1/3
  In3/1 -> Switch1/1
  Switch1/1 -> Out2/1
  In6/1 -> Switch2/3
  In5/1 -> Switch2/1
  In8/1 -> Switch3/3
  In7/1 -> Switch3/1
  Switch2/1 -> Out3/1
  Switch3/1 -> Out4/1

== system SGBMDisparityExample_original/SGBMHDLAlgorithm/PostProcessing/Interpolation/Minimum_Cost_Index/For Each Subsystem2 ==
  In1 : Inport  Partition=on  PartitionDimension=1  PartitionWidth=1  PartitionOffset=0
  In2 : Inport  Port=2  Partition=on  PartitionDimension=1  PartitionWidth=1  PartitionOffset=0
  In3 : Inport  Port=3  Partition=on  PartitionDimension=1  PartitionWidth=1  PartitionOffset=0
  In4 : Inport  Port=4  Partition=on  PartitionDimension=1  PartitionWidth=1  PartitionOffset=0
  In5 : Inport  Port=5  Partition=on  PartitionDimension=1  PartitionWidth=1  PartitionOffset=0
  In6 : Inport  Port=6  Partition=on  PartitionDimension=1  PartitionWidth=1  PartitionOffset=0
  In7 : Inport  Port=7  Partition=on  PartitionDimension=1  PartitionWidth=1  PartitionOffset=0
  In8 : Inport  Port=8  Partition=on  PartitionDimension=1  PartitionWidth=1  PartitionOffset=0
  For Each : ForEach  DisableCoverage=on
  Relational Operator : RelationalOperator  Operator=<=  OutDataTypeStr=boolean  RndMeth=Nearest
  Switch{,1..3} (4 alike) : Switch  Criteria=u2 ~= 0
  Out1 : Outport  ConcatenationDimension=1  VectorParamsAs1DForOutWhenUnconnected=off
  Out2 : Outport  Port=2  ConcatenationDimension=1  VectorParamsAs1DForOutWhenUnconnected=off
  Out3 : Outport  Port=3  ConcatenationDimension=1  VectorParamsAs1DForOutWhenUnconnected=off
  Out4 : Outport  Port=4  ConcatenationDimension=1  VectorParamsAs1DForOutWhenUnconnected=off
  wires:
  In1/1 -> Relational Operator/1, Switch/1
  In2/1 -> Relational Operator/2, Switch/3
  Relational Operator/1 -> Switch3/2, Switch2/2, Switch1/2, Switch/2
  Switch/1 -> Out1/1
  In4/1 -> Switch1/3
  In3/1 -> Switch1/1
  Switch1/1 -> Out2/1
  In6/1 -> Switch2/3
  In5/1 -> Switch2/1
  In8/1 -> Switch3/3
  In7/1 -> Switch3/1
  Switch2/1 -> Out3/1
  Switch3/1 -> Out4/1

== system SGBMDisparityExample_original/SGBMHDLAlgorithm/PostProcessing/Interpolation/Minimum_Cost_Index/For Each Subsystem3 ==
  In1 : Inport  Partition=on  PartitionDimension=1  PartitionWidth=1  PartitionOffset=0
  In2 : Inport  Port=2  Partition=on  PartitionDimension=1  PartitionWidth=1  PartitionOffset=0
  In3 : Inport  Port=3  Partition=on  PartitionDimension=1  PartitionWidth=1  PartitionOffset=0
  In4 : Inport  Port=4  Partition=on  PartitionDimension=1  PartitionWidth=1  PartitionOffset=0
  In5 : Inport  Port=5  Partition=on  PartitionDimension=1  PartitionWidth=1  PartitionOffset=0
  In6 : Inport  Port=6  Partition=on  PartitionDimension=1  PartitionWidth=1  PartitionOffset=0
  In7 : Inport  Port=7  Partition=on  PartitionDimension=1  PartitionWidth=1  PartitionOffset=0
  In8 : Inport  Port=8  Partition=on  PartitionDimension=1  PartitionWidth=1  PartitionOffset=0
  For Each : ForEach  DisableCoverage=on
  Relational Operator : RelationalOperator  Operator=<=  OutDataTypeStr=boolean  RndMeth=Nearest
  Switch{,1..3} (4 alike) : Switch  Criteria=u2 ~= 0
  Out1 : Outport  ConcatenationDimension=1  VectorParamsAs1DForOutWhenUnconnected=off
  Out2 : Outport  Port=2  ConcatenationDimension=1  VectorParamsAs1DForOutWhenUnconnected=off
  Out3 : Outport  Port=3  ConcatenationDimension=1  VectorParamsAs1DForOutWhenUnconnected=off
  Out4 : Outport  Port=4  ConcatenationDimension=1  VectorParamsAs1DForOutWhenUnconnected=off
  wires:
  In1/1 -> Relational Operator/1, Switch/1
  In2/1 -> Relational Operator/2, Switch/3
  Relational Operator/1 -> Switch3/2, Switch2/2, Switch1/2, Switch/2
  Switch/1 -> Out1/1
  In4/1 -> Switch1/3
  In3/1 -> Switch1/1
  Switch1/1 -> Out2/1
  In6/1 -> Switch2/3
  In5/1 -> Switch2/1
  In8/1 -> Switch3/3
  In7/1 -> Switch3/1
  Switch2/1 -> Out3/1
  Switch3/1 -> Out4/1

== system SGBMDisparityExample_original/SGBMHDLAlgorithm/PostProcessing/Interpolation/Minimum_Cost_Index/For Each Subsystem4 ==
  In1 : Inport  Partition=on  PartitionDimension=1  PartitionWidth=1  PartitionOffset=0
  In2 : Inport  Port=2  Partition=on  PartitionDimension=1  PartitionWidth=1  PartitionOffset=0
  In3 : Inport  Port=3  Partition=on  PartitionDimension=1  PartitionWidth=1  PartitionOffset=0
  In4 : Inport  Port=4  Partition=on  PartitionDimension=1  PartitionWidth=1  PartitionOffset=0
  In5 : Inport  Port=5  Partition=on  PartitionDimension=1  PartitionWidth=1  PartitionOffset=0
  In6 : Inport  Port=6  Partition=on  PartitionDimension=1  PartitionWidth=1  PartitionOffset=0
  In7 : Inport  Port=7  Partition=on  PartitionDimension=1  PartitionWidth=1  PartitionOffset=0
  In8 : Inport  Port=8  Partition=on  PartitionDimension=1  PartitionWidth=1  PartitionOffset=0
  For Each : ForEach  DisableCoverage=on
  Relational Operator : RelationalOperator  Operator=<=  OutDataTypeStr=boolean  RndMeth=Nearest
  Switch{,1..3} (4 alike) : Switch  Criteria=u2 ~= 0
  Out1 : Outport  ConcatenationDimension=1  VectorParamsAs1DForOutWhenUnconnected=off
  Out2 : Outport  Port=2  ConcatenationDimension=1  VectorParamsAs1DForOutWhenUnconnected=off
  Out3 : Outport  Port=3  ConcatenationDimension=1  VectorParamsAs1DForOutWhenUnconnected=off
  Out4 : Outport  Port=4  ConcatenationDimension=1  VectorParamsAs1DForOutWhenUnconnected=off
  wires:
  In1/1 -> Relational Operator/1, Switch/1
  In2/1 -> Relational Operator/2, Switch/3
  Relational Operator/1 -> Switch3/2, Switch2/2, Switch1/2, Switch/2
  Switch/1 -> Out1/1
  In4/1 -> Switch1/3
  In3/1 -> Switch1/1
  Switch1/1 -> Out2/1
  In6/1 -> Switch2/3
  In5/1 -> Switch2/1
  In8/1 -> Switch3/3
  In7/1 -> Switch3/1
  Switch2/1 -> Out3/1
  Switch3/1 -> Out4/1

== system SGBMDisparityExample_original/SGBMHDLAlgorithm/PostProcessing/Interpolation/Minimum_Cost_Index/For Each Subsystem5 ==
  In1 : Inport  Partition=on  PartitionDimension=1  PartitionWidth=1  PartitionOffset=0
  In2 : Inport  Port=2  Partition=on  PartitionDimension=1  PartitionWidth=1  PartitionOffset=0
  In3 : Inport  Port=3  Partition=on  PartitionDimension=1  PartitionWidth=1  PartitionOffset=0
  In4 : Inport  Port=4  Partition=on  PartitionDimension=1  PartitionWidth=1  PartitionOffset=0
  In5 : Inport  Port=5  Partition=on  PartitionDimension=1  PartitionWidth=1  PartitionOffset=0
  In6 : Inport  Port=6  Partition=on  PartitionDimension=1  PartitionWidth=1  PartitionOffset=0
  In7 : Inport  Port=7  Partition=on  PartitionDimension=1  PartitionWidth=1  PartitionOffset=0
  In8 : Inport  Port=8  Partition=on  PartitionDimension=1  PartitionWidth=1  PartitionOffset=0
  For Each : ForEach  DisableCoverage=on
  Relational Operator : RelationalOperator  Operator=<=  OutDataTypeStr=boolean  RndMeth=Nearest
  Switch{,1..3} (4 alike) : Switch  Criteria=u2 ~= 0
  Out1 : Outport  ConcatenationDimension=1  VectorParamsAs1DForOutWhenUnconnected=off
  Out2 : Outport  Port=2  ConcatenationDimension=1  VectorParamsAs1DForOutWhenUnconnected=off
  Out3 : Outport  Port=3  ConcatenationDimension=1  VectorParamsAs1DForOutWhenUnconnected=off
  Out4 : Outport  Port=4  ConcatenationDimension=1  VectorParamsAs1DForOutWhenUnconnected=off
  wires:
  In1/1 -> Relational Operator/1, Switch/1
  In2/1 -> Relational Operator/2, Switch/3
  Relational Operator/1 -> Switch3/2, Switch2/2, Switch1/2, Switch/2
  Switch/1 -> Out1/1
  In4/1 -> Switch1/3
  In3/1 -> Switch1/1
  Switch1/1 -> Out2/1
  In6/1 -> Switch2/3
  In5/1 -> Switch2/1
  In8/1 -> Switch3/3
  In7/1 -> Switch3/1
  Switch2/1 -> Out3/1
  Switch3/1 -> Out4/1

== system SGBMDisparityExample_original/SGBMHDLAlgorithm/PostProcessing/Interpolation/Minimum_Cost_Index/For Each Subsystem6 ==
  In1 : Inport  Partition=on  PartitionDimension=1  PartitionWidth=1  PartitionOffset=0
  In2 : Inport  Port=2  Partition=on  PartitionDimension=1  PartitionWidth=1  PartitionOffset=0
  In3 : Inport  Port=3  Partition=on  PartitionDimension=1  PartitionWidth=1  PartitionOffset=0
  In4 : Inport  Port=4  Partition=on  PartitionDimension=1  PartitionWidth=1  PartitionOffset=0
  In5 : Inport  Port=5  Partition=on  PartitionDimension=1  PartitionWidth=1  PartitionOffset=0
  In6 : Inport  Port=6  Partition=on  PartitionDimension=1  PartitionWidth=1  PartitionOffset=0
  In7 : Inport  Port=7  Partition=on  PartitionDimension=1  PartitionWidth=1  PartitionOffset=0
  In8 : Inport  Port=8  Partition=on  PartitionDimension=1  PartitionWidth=1  PartitionOffset=0
  For Each : ForEach  DisableCoverage=on
  Relational Operator : RelationalOperator  Operator=<=  OutDataTypeStr=boolean  RndMeth=Nearest
  Switch{,1..3} (4 alike) : Switch  Criteria=u2 ~= 0
  Out1 : Outport  ConcatenationDimension=1  VectorParamsAs1DForOutWhenUnconnected=off
  Out2 : Outport  Port=2  ConcatenationDimension=1  VectorParamsAs1DForOutWhenUnconnected=off
  Out3 : Outport  Port=3  ConcatenationDimension=1  VectorParamsAs1DForOutWhenUnconnected=off
  Out4 : Outport  Port=4  ConcatenationDimension=1  VectorParamsAs1DForOutWhenUnconnected=off
  wires:
  In1/1 -> Relational Operator/1, Switch/1
  In2/1 -> Relational Operator/2, Switch/3
  Relational Operator/1 -> Switch3/2, Switch2/2, Switch1/2, Switch/2
  Switch/1 -> Out1/1
  In4/1 -> Switch1/3
  In3/1 -> Switch1/1
  Switch1/1 -> Out2/1
  In6/1 -> Switch2/3
  In5/1 -> Switch2/1
  In8/1 -> Switch3/3
  In7/1 -> Switch3/1
  Switch2/1 -> Out3/1
  Switch3/1 -> Out4/1

== system SGBMDisparityExample_original/SGBMHDLAlgorithm/PostProcessing/Interpolation/Division/QuoRem/First ==
  In1 : Inport
  In2 : Inport  Port=2
  Add : Sum  OutDataTypeStr=fixdt(0,13,0)
  Add1 : Sum  Inputs=+-  OutDataTypeStr=fixdt(0,13,0)
  Bit Concat2 : hdlsllib/Logic and Bit Operations/Bit Concat  numInputs=2
  Bit Shift : hdlsllib/Logic and Bit Operations/Bit Shift  mode=Shift Left Logical  N=1
  Bitwise Operator : simulink/Logic and Bit Operations/Bitwise Operator  logicop=OR  UseBitMask=on  BitMask=bin2dec('0')  BitMaskRealWorld=Stored Integer
  Bitwise Operator2 : simulink/Logic and Bit Operations/Bitwise Operator  logicop=OR  UseBitMask=on  BitMask=bin2dec('1')  BitMaskRealWorld=Stored Integer
  Extract Bits1 : simulink/Logic and Bit Operations/Extract Bits  bitsToExtract=Range starting with most significant bit  numBits=1  bitIdxRange=[7]  outScalingMode=Treat bit field as an integer
  Extract Bits2 : simulink/Logic and Bit Operations/Extract Bits  bitsToExtract=Range starting with most significant bit  numBits=1  bitIdxRange=[7]  outScalingMode=Treat bit field as an integer
  Extract Bits3 : simulink/Logic and Bit Operations/Extract Bits  bitsToExtract=Upper half  numBits=8  bitIdxRange=[7]  outScalingMode=Treat bit field as an integer
  Extract Bits4 : simulink/Logic and Bit Operations/Extract Bits  bitsToExtract=Lower half  numBits=8  bitIdxRange=[7]  outScalingMode=Treat bit field as an integer
  Extract Bits5 : simulink/Logic and Bit Operations/Extract Bits  bitsToExtract=Range starting with most significant bit  numBits=1  bitIdxRange=[7]  outScalingMode=Treat bit field as an integer
  Switch : Switch  Criteria=u2 ~= 0
  Switch1 : Switch  Criteria=u2 ~= 0
  Switch2 : Switch  Criteria=u2 ~= 0
  Out1 : Outport  VectorParamsAs1DForOutWhenUnconnected=off
  Out2 : Outport  Port=2  VectorParamsAs1DForOutWhenUnconnected=off
  Start : Outport  Port=3  VectorParamsAs1DForOutWhenUnconnected=off
  wires:
  Add/1 -> Switch/1
  Bitwise Operator2/1 -> Switch1/3
  Bitwise Operator/1 -> Switch1/1
  Extract Bits2/1 -> Switch1/2
  Add1/1 -> Switch/3
  In1/1 -> Extract Bits1/1, Bit Shift/1
  Extract Bits3/1 -> Add1/1, Add/1
  Bit Concat2/1 -> Switch2/1
  Extract Bits1/1 -> Switch/2
  Extract Bits4/1 -> Bitwise Operator2/1, Bitwise Operator/1, Extract Bits5/1
  Switch1/1 -> Bit Concat2/2
  Switch/1 -> Bit Concat2/1, Extract Bits2/1
  Switch2/1 -> Out1/1
  Bit Shift/1 -> Switch2/3, Extract Bits4/1, Extract Bits3/1
  Extract Bits5/1 -> Start/1, Switch2/2
  In2/1 -> Out2/1, Add1/2, Add/2
